simulink model "kadai3_PI"  (R2019b)
settings: Solver=VariableStepAuto  StartTime=0.0  StopTime=10.0  RelTol=1e-3
values from neighbouring files (symbols this model uses):
  D = 1    [ex01.m]
  J = 1    [ex01.m]
  Kiv = 1    [ex01.m]
  Kpv = 1    [ex01.m]
  Kt = 1    [ex01.m]
settings Model: Creator=ryoga  LastModifiedBy=ryoga

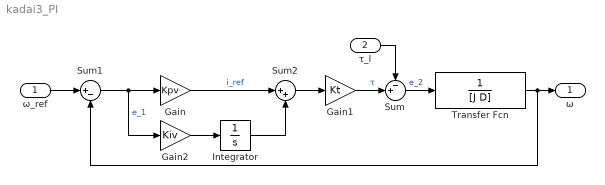
== system kadai3_PI ==
  ω_ref : Inport
  τ_l : Inport  Port=2
  Gain : Gain  Gain=Kpv
  Gain1 : Gain  Gain=Kt
  Gain2 : Gain  Gain=Kiv
  Integrator : Integrator
  Sum : Sum  Inputs=-+|
  Sum1 : Sum  Inputs=|+-
  Sum2 : Sum  Inputs=|++
  Transfer Fcn : TransferFcn  Denominator=[J D]
  ω : Outport
  wires:
  Sum/1 -> Transfer Fcn/1  "e_2"
  τ_l/1 -> Sum/1
  Transfer Fcn/1 -> Sum1/2, ω/1
  Gain1/1 -> Sum/2  "τ"
  ω_ref/1 -> Sum1/1
  Sum1/1 -> Gain2/1, Gain/1  "e_1"
  Gain2/1 -> Integrator/1
  Sum2/1 -> Gain1/1
  Integrator/1 -> Sum2/2
  Gain/1 -> Sum2/1  "i_ref"
